simulink model "Microgrid_W"  (R2020a)
settings: Solver=ode15s  StartTime=0  StopTime=1440*1  MaxStep=1  RelTol=1e-3
libraries: simulink x4214, powerlib x685, simulink_extras x28, Microgrid_Library x18, powerlib_meascontrol x12
(part 38 of 48)

== system Microgrid_W/House 5 W1/Light 2/D10 ==
  Add : Sum  Inputs=+++
  Clock : Clock
  Compare To Zero : simulink/Logic and Bit Operations/Compare To Zero  relop=>  OutDataTypeStr=boolean
  Compare To Zero1 : simulink/Logic and Bit Operations/Compare To Zero  relop=>  OutDataTypeStr=boolean
  Compare To Zero2 : simulink/Logic and Bit Operations/Compare To Zero  relop=>  OutDataTypeStr=boolean
  Constant : Constant
  Constant{1..2,5,8} (4 alike) : Constant  Value=0
  Constant3 : Constant  Value=Dishwasher_On
  Constant4 : Constant
  Constant6 : Constant  Value=Dishwasher_On
  Constant7 : Constant
  Constant9 : Constant  Value=Dishwasher_On
  Gain : Gain  Gain=t
  Interval Test : simulink/Logic and Bit Operations/Interval Test  IntervalClosedRight=on  uplimit=Dishwasher_On+89+86400*2  IntervalClosedLeft=on  lowlimit=Dishwasher_On+82+86400*2  OutDataTypeStr=boolean
  Interval Test1 : simulink/Logic and Bit Operations/Interval Test  IntervalClosedRight=on  uplimit=Dishwasher_On+95+86400*2  IntervalClosedLeft=on  lowlimit=Dishwasher_On+90+86400*2  OutDataTypeStr=boolean
  Interval Test2 : simulink/Logic and Bit Operations/Interval Test  IntervalClosedRight=on  uplimit=Dishwasher_On+102+86400*2  IntervalClosedLeft=on  lowlimit=Dishwasher_On+97+86400*2  OutDataTypeStr=boolean
  Switch{,1..5} (6 alike) : Switch  Criteria=u2 > Threshold  Threshold=0.5
  Out1 : Outport  VectorParamsAs1DForOutWhenUnconnected=off
  wires:
  Clock/1 -> Gain/1
  Add/1 -> Out1/1
  Switch3/1 -> Add/3
  Switch2/1 -> Add/2
  Switch/1 -> Add/1
  Switch5/1 -> Switch3/1
  Switch4/1 -> Switch2/1
  Compare To Zero2/1 -> Switch5/2
  Constant8/1 -> Switch5/3
  Constant7/1 -> Switch5/1
  Constant9/1 -> Compare To Zero2/1
  Compare To Zero1/1 -> Switch4/2
  Constant5/1 -> Switch4/3
  Constant4/1 -> Switch4/1
  Constant6/1 -> Compare To Zero1/1
  Interval Test2/1 -> Switch3/2
  Interval Test1/1 -> Switch2/2
  Switch1/1 -> Switch/1
  Compare To Zero/1 -> Switch1/2
  Constant2/1 -> Switch1/3
  Constant/1 -> Switch1/1
  Constant3/1 -> Compare To Zero/1
  Gain/1 -> Interval Test/1, Interval Test1/1, Interval Test2/1
  Constant1/1 -> Switch/3, Switch2/3, Switch3/3
  Interval Test/1 -> Switch/2

== system Microgrid_W/House 5 W1/Light 2/D11 ==
  Add : Sum  Inputs=+++
  Clock : Clock
  Compare To Zero : simulink/Logic and Bit Operations/Compare To Zero  relop=>  OutDataTypeStr=boolean
  Compare To Zero1 : simulink/Logic and Bit Operations/Compare To Zero  relop=>  OutDataTypeStr=boolean
  Compare To Zero2 : simulink/Logic and Bit Operations/Compare To Zero  relop=>  OutDataTypeStr=boolean
  Constant : Constant
  Constant{1..2,5,8} (4 alike) : Constant  Value=0
  Constant3 : Constant  Value=Dishwasher_On
  Constant4 : Constant
  Constant6 : Constant  Value=Dishwasher_On
  Constant7 : Constant
  Constant9 : Constant  Value=Dishwasher_On
  Gain : Gain  Gain=t
  Interval Test : simulink/Logic and Bit Operations/Interval Test  IntervalClosedRight=on  uplimit=Dishwasher_On+89+86400*3  IntervalClosedLeft=on  lowlimit=Dishwasher_On+82+86400*3  OutDataTypeStr=boolean
  Interval Test1 : simulink/Logic and Bit Operations/Interval Test  IntervalClosedRight=on  uplimit=Dishwasher_On+95+86400*3  IntervalClosedLeft=on  lowlimit=Dishwasher_On+90+86400*3  OutDataTypeStr=boolean
  Interval Test2 : simulink/Logic and Bit Operations/Interval Test  IntervalClosedRight=on  uplimit=Dishwasher_On+102+86400*3  IntervalClosedLeft=on  lowlimit=Dishwasher_On+97+86400*3  OutDataTypeStr=boolean
  Switch{,1..5} (6 alike) : Switch  Criteria=u2 > Threshold  Threshold=0.5
  Out1 : Outport  VectorParamsAs1DForOutWhenUnconnected=off
  wires:
  Clock/1 -> Gain/1
  Interval Test/1 -> Switch/2
  Constant1/1 -> Switch3/3, Switch2/3, Switch/3
  Gain/1 -> Interval Test2/1, Interval Test1/1, Interval Test/1
  Constant3/1 -> Compare To Zero/1
  Constant/1 -> Switch1/1
  Constant2/1 -> Switch1/3
  Compare To Zero/1 -> Switch1/2
  Switch1/1 -> Switch/1
  Interval Test1/1 -> Switch2/2
  Interval Test2/1 -> Switch3/2
  Constant6/1 -> Compare To Zero1/1
  Constant4/1 -> Switch4/1
  Constant5/1 -> Switch4/3
  Compare To Zero1/1 -> Switch4/2
  Constant9/1 -> Compare To Zero2/1
  Constant7/1 -> Switch5/1
  Constant8/1 -> Switch5/3
  Compare To Zero2/1 -> Switch5/2
  Switch4/1 -> Switch2/1
  Switch5/1 -> Switch3/1
  Switch/1 -> Add/1
  Switch2/1 -> Add/2
  Switch3/1 -> Add/3
  Add/1 -> Out1/1

== system Microgrid_W/House 5 W1/Light 2/D12 ==
  Add : Sum  Inputs=+++
  Clock : Clock
  Compare To Zero : simulink/Logic and Bit Operations/Compare To Zero  relop=>  OutDataTypeStr=boolean
  Compare To Zero1 : simulink/Logic and Bit Operations/Compare To Zero  relop=>  OutDataTypeStr=boolean
  Compare To Zero2 : simulink/Logic and Bit Operations/Compare To Zero  relop=>  OutDataTypeStr=boolean
  Constant : Constant
  Constant{1..2,5,8} (4 alike) : Constant  Value=0
  Constant3 : Constant  Value=Dishwasher_On
  Constant4 : Constant
  Constant6 : Constant  Value=Dishwasher_On
  Constant7 : Constant
  Constant9 : Constant  Value=Dishwasher_On
  Gain : Gain  Gain=t
  Interval Test : simulink/Logic and Bit Operations/Interval Test  IntervalClosedRight=on  uplimit=Dishwasher_On+89+86400*4  IntervalClosedLeft=on  lowlimit=Dishwasher_On+82+86400*4  OutDataTypeStr=boolean
  Interval Test1 : simulink/Logic and Bit Operations/Interval Test  IntervalClosedRight=on  uplimit=Dishwasher_On+95+86400*4  IntervalClosedLeft=on  lowlimit=Dishwasher_On+90+86400*4  OutDataTypeStr=boolean
  Interval Test2 : simulink/Logic and Bit Operations/Interval Test  IntervalClosedRight=on  uplimit=Dishwasher_On+102+86400*4  IntervalClosedLeft=on  lowlimit=Dishwasher_On+97+86400*4  OutDataTypeStr=boolean
  Switch{,1..5} (6 alike) : Switch  Criteria=u2 > Threshold  Threshold=0.5
  Out1 : Outport  VectorParamsAs1DForOutWhenUnconnected=off
  wires:
  Clock/1 -> Gain/1
  Add/1 -> Out1/1
  Switch3/1 -> Add/3
  Switch2/1 -> Add/2
  Switch/1 -> Add/1
  Switch5/1 -> Switch3/1
  Switch4/1 -> Switch2/1
  Compare To Zero2/1 -> Switch5/2
  Constant8/1 -> Switch5/3
  Constant7/1 -> Switch5/1
  Constant9/1 -> Compare To Zero2/1
  Compare To Zero1/1 -> Switch4/2
  Constant5/1 -> Switch4/3
  Constant4/1 -> Switch4/1
  Constant6/1 -> Compare To Zero1/1
  Interval Test2/1 -> Switch3/2
  Interval Test1/1 -> Switch2/2
  Switch1/1 -> Switch/1
  Compare To Zero/1 -> Switch1/2
  Constant2/1 -> Switch1/3
  Constant/1 -> Switch1/1
  Constant3/1 -> Compare To Zero/1
  Gain/1 -> Interval Test/1, Interval Test1/1, Interval Test2/1
  Constant1/1 -> Switch/3, Switch2/3, Switch3/3
  Interval Test/1 -> Switch/2

== system Microgrid_W/House 5 W1/Light 2/D13 ==
  Add : Sum  Inputs=+++
  Clock : Clock
  Compare To Zero : simulink/Logic and Bit Operations/Compare To Zero  relop=>  OutDataTypeStr=boolean
  Compare To Zero1 : simulink/Logic and Bit Operations/Compare To Zero  relop=>  OutDataTypeStr=boolean
  Compare To Zero2 : simulink/Logic and Bit Operations/Compare To Zero  relop=>  OutDataTypeStr=boolean
  Constant : Constant
  Constant{1..2,5,8} (4 alike) : Constant  Value=0
  Constant3 : Constant  Value=Dishwasher_On
  Constant4 : Constant
  Constant6 : Constant  Value=Dishwasher_On
  Constant7 : Constant
  Constant9 : Constant  Value=Dishwasher_On
  Gain : Gain  Gain=t
  Interval Test : simulink/Logic and Bit Operations/Interval Test  IntervalClosedRight=on  uplimit=Dishwasher_On+89+86400*5  IntervalClosedLeft=on  lowlimit=Dishwasher_On+82+86400*5  OutDataTypeStr=boolean
  Interval Test1 : simulink/Logic and Bit Operations/Interval Test  IntervalClosedRight=on  uplimit=Dishwasher_On+95+86400*5  IntervalClosedLeft=on  lowlimit=Dishwasher_On+90+86400*5  OutDataTypeStr=boolean
  Interval Test2 : simulink/Logic and Bit Operations/Interval Test  IntervalClosedRight=on  uplimit=Dishwasher_On+102+86400*5  IntervalClosedLeft=on  lowlimit=Dishwasher_On+97+86400*5  OutDataTypeStr=boolean
  Switch{,1..5} (6 alike) : Switch  Criteria=u2 > Threshold  Threshold=0.5
  Out1 : Outport  VectorParamsAs1DForOutWhenUnconnected=off
  wires:
  Clock/1 -> Gain/1
  Interval Test/1 -> Switch/2
  Constant1/1 -> Switch3/3, Switch2/3, Switch/3
  Gain/1 -> Interval Test2/1, Interval Test1/1, Interval Test/1
  Constant3/1 -> Compare To Zero/1
  Constant/1 -> Switch1/1
  Constant2/1 -> Switch1/3
  Compare To Zero/1 -> Switch1/2
  Switch1/1 -> Switch/1
  Interval Test1/1 -> Switch2/2
  Interval Test2/1 -> Switch3/2
  Constant6/1 -> Compare To Zero1/1
  Constant4/1 -> Switch4/1
  Constant5/1 -> Switch4/3
  Compare To Zero1/1 -> Switch4/2
  Constant9/1 -> Compare To Zero2/1
  Constant7/1 -> Switch5/1
  Constant8/1 -> Switch5/3
  Compare To Zero2/1 -> Switch5/2
  Switch4/1 -> Switch2/1
  Switch5/1 -> Switch3/1
  Switch/1 -> Add/1
  Switch2/1 -> Add/2
  Switch3/1 -> Add/3
  Add/1 -> Out1/1

== system Microgrid_W/House 5 W1/Light 2/D14 ==
  Add : Sum  Inputs=+++
  Clock : Clock
  Compare To Zero : simulink/Logic and Bit Operations/Compare To Zero  relop=>  OutDataTypeStr=boolean
  Compare To Zero1 : simulink/Logic and Bit Operations/Compare To Zero  relop=>  OutDataTypeStr=boolean
  Compare To Zero2 : simulink/Logic and Bit Operations/Compare To Zero  relop=>  OutDataTypeStr=boolean
  Constant : Constant
  Constant{1..2,5,8} (4 alike) : Constant  Value=0
  Constant3 : Constant  Value=Dishwasher_On
  Constant4 : Constant
  Constant6 : Constant  Value=Dishwasher_On
  Constant7 : Constant
  Constant9 : Constant  Value=Dishwasher_On
  Gain : Gain  Gain=t
  Interval Test : simulink/Logic and Bit Operations/Interval Test  IntervalClosedRight=on  uplimit=Dishwasher_On+89+86400*6  IntervalClosedLeft=on  lowlimit=Dishwasher_On+82+86400*6  OutDataTypeStr=boolean
  Interval Test1 : simulink/Logic and Bit Operations/Interval Test  IntervalClosedRight=on  uplimit=Dishwasher_On+95+86400*6  IntervalClosedLeft=on  lowlimit=Dishwasher_On+90+86400*6  OutDataTypeStr=boolean
  Interval Test2 : simulink/Logic and Bit Operations/Interval Test  IntervalClosedRight=on  uplimit=Dishwasher_On+102+86400*6  IntervalClosedLeft=on  lowlimit=Dishwasher_On+97+86400*6  OutDataTypeStr=boolean
  Switch{,1..5} (6 alike) : Switch  Criteria=u2 > Threshold  Threshold=0.5
  Out1 : Outport  VectorParamsAs1DForOutWhenUnconnected=off
  wires:
  Clock/1 -> Gain/1
  Add/1 -> Out1/1
  Switch3/1 -> Add/3
  Switch2/1 -> Add/2
  Switch/1 -> Add/1
  Switch5/1 -> Switch3/1
  Switch4/1 -> Switch2/1
  Compare To Zero2/1 -> Switch5/2
  Constant8/1 -> Switch5/3
  Constant7/1 -> Switch5/1
  Constant9/1 -> Compare To Zero2/1
  Compare To Zero1/1 -> Switch4/2
  Constant5/1 -> Switch4/3
  Constant4/1 -> Switch4/1
  Constant6/1 -> Compare To Zero1/1
  Interval Test2/1 -> Switch3/2
  Interval Test1/1 -> Switch2/2
  Switch1/1 -> Switch/1
  Compare To Zero/1 -> Switch1/2
  Constant2/1 -> Switch1/3
  Constant/1 -> Switch1/1
  Constant3/1 -> Compare To Zero/1
  Gain/1 -> Interval Test/1, Interval Test1/1, Interval Test2/1
  Constant1/1 -> Switch/3, Switch2/3, Switch3/3
  Interval Test/1 -> Switch/2

== system Microgrid_W/House 5 W1/Light 2/D15 ==
  Add : Sum  Inputs=+++
  Clock : Clock
  Compare To Zero : simulink/Logic and Bit Operations/Compare To Zero  relop=>  OutDataTypeStr=boolean
  Compare To Zero1 : simulink/Logic and Bit Operations/Compare To Zero  relop=>  OutDataTypeStr=boolean
  Compare To Zero2 : simulink/Logic and Bit Operations/Compare To Zero  relop=>  OutDataTypeStr=boolean
  Constant : Constant
  Constant{1..2,5,8} (4 alike) : Constant  Value=0
  Constant3 : Constant  Value=Dishwasher_On
  Constant4 : Constant
  Constant6 : Constant  Value=Dishwasher_On
  Constant7 : Constant
  Constant9 : Constant  Value=Dishwasher_On
  Gain : Gain  Gain=t
  Interval Test : simulink/Logic and Bit Operations/Interval Test  IntervalClosedRight=on  uplimit=Dishwasher_On+10  IntervalClosedLeft=on  lowlimit=Dishwasher_On  OutDataTypeStr=boolean
  Interval Test1 : simulink/Logic and Bit Operations/Interval Test  IntervalClosedRight=on  uplimit=Dishwasher_On+48  IntervalClosedLeft=on  lowlimit=Dishwasher_On+23  OutDataTypeStr=boolean
  Interval Test2 : simulink/Logic and Bit Operations/Interval Test  IntervalClosedRight=on  uplimit=Dishwasher_On+75  IntervalClosedLeft=on  lowlimit=Dishwasher_On+66  OutDataTypeStr=boolean
  Switch{,1..5} (6 alike) : Switch  Criteria=u2 > Threshold  Threshold=0.5
  Out1 : Outport  VectorParamsAs1DForOutWhenUnconnected=off
  wires:
  Clock/1 -> Gain/1
  Interval Test/1 -> Switch/2
  Constant1/1 -> Switch3/3, Switch2/3, Switch/3
  Gain/1 -> Interval Test2/1, Interval Test1/1, Interval Test/1
  Constant3/1 -> Compare To Zero/1
  Constant/1 -> Switch1/1
  Constant2/1 -> Switch1/3
  Compare To Zero/1 -> Switch1/2
  Switch1/1 -> Switch/1
  Interval Test1/1 -> Switch2/2
  Interval Test2/1 -> Switch3/2
  Constant6/1 -> Compare To Zero1/1
  Constant4/1 -> Switch4/1
  Constant5/1 -> Switch4/3
  Compare To Zero1/1 -> Switch4/2
  Constant9/1 -> Compare To Zero2/1
  Constant7/1 -> Switch5/1
  Constant8/1 -> Switch5/3
  Compare To Zero2/1 -> Switch5/2
  Switch4/1 -> Switch2/1
  Switch5/1 -> Switch3/1
  Switch/1 -> Add/1
  Switch2/1 -> Add/2
  Switch3/1 -> Add/3
  Add/1 -> Out1/1

== system Microgrid_W/House 5 W1/Light 2/D16 ==
  Add : Sum  Inputs=+++
  Clock : Clock
  Compare To Zero : simulink/Logic and Bit Operations/Compare To Zero  relop=>  OutDataTypeStr=boolean
  Compare To Zero1 : simulink/Logic and Bit Operations/Compare To Zero  relop=>  OutDataTypeStr=boolean
  Compare To Zero2 : simulink/Logic and Bit Operations/Compare To Zero  relop=>  OutDataTypeStr=boolean
  Constant : Constant
  Constant{1..2,5,8} (4 alike) : Constant  Value=0
  Constant3 : Constant  Value=Dishwasher_On
  Constant4 : Constant
  Constant6 : Constant  Value=Dishwasher_On
  Constant7 : Constant
  Constant9 : Constant  Value=Dishwasher_On
  Gain : Gain  Gain=t
  Interval Test : simulink/Logic and Bit Operations/Interval Test  IntervalClosedRight=on  uplimit=Dishwasher_On+10+86400  IntervalClosedLeft=on  lowlimit=Dishwasher_On+86400  OutDataTypeStr=boolean
  Interval Test1 : simulink/Logic and Bit Operations/Interval Test  IntervalClosedRight=on  uplimit=Dishwasher_On+48+86400  IntervalClosedLeft=on  lowlimit=Dishwasher_On+23+86400  OutDataTypeStr=boolean
  Interval Test2 : simulink/Logic and Bit Operations/Interval Test  IntervalClosedRight=on  uplimit=Dishwasher_On+75+86400  IntervalClosedLeft=on  lowlimit=Dishwasher_On+66+86400  OutDataTypeStr=boolean
  Switch{,1..5} (6 alike) : Switch  Criteria=u2 > Threshold  Threshold=0.5
  Out1 : Outport  VectorParamsAs1DForOutWhenUnconnected=off
  wires:
  Clock/1 -> Gain/1
  Add/1 -> Out1/1
  Switch3/1 -> Add/3
  Switch2/1 -> Add/2
  Switch/1 -> Add/1
  Switch5/1 -> Switch3/1
  Switch4/1 -> Switch2/1
  Compare To Zero2/1 -> Switch5/2
  Constant8/1 -> Switch5/3
  Constant7/1 -> Switch5/1
  Constant9/1 -> Compare To Zero2/1
  Compare To Zero1/1 -> Switch4/2
  Constant5/1 -> Switch4/3
  Constant4/1 -> Switch4/1
  Constant6/1 -> Compare To Zero1/1
  Interval Test2/1 -> Switch3/2
  Interval Test1/1 -> Switch2/2
  Switch1/1 -> Switch/1
  Compare To Zero/1 -> Switch1/2
  Constant2/1 -> Switch1/3
  Constant/1 -> Switch1/1
  Constant3/1 -> Compare To Zero/1
  Gain/1 -> Interval Test/1, Interval Test1/1, Interval Test2/1
  Constant1/1 -> Switch/3, Switch2/3, Switch3/3
  Interval Test/1 -> Switch/2

== system Microgrid_W/House 5 W1/Light 2/D17 ==
  Add : Sum  Inputs=+++
  Clock : Clock
  Compare To Zero : simulink/Logic and Bit Operations/Compare To Zero  relop=>  OutDataTypeStr=boolean
  Compare To Zero1 : simulink/Logic and Bit Operations/Compare To Zero  relop=>  OutDataTypeStr=boolean
  Compare To Zero2 : simulink/Logic and Bit Operations/Compare To Zero  relop=>  OutDataTypeStr=boolean
  Constant : Constant
  Constant{1..2,5,8} (4 alike) : Constant  Value=0
  Constant3 : Constant  Value=Dishwasher_On
  Constant4 : Constant
  Constant6 : Constant  Value=Dishwasher_On
  Constant7 : Constant
  Constant9 : Constant  Value=Dishwasher_On
  Gain : Gain  Gain=t
  Interval Test : simulink/Logic and Bit Operations/Interval Test  IntervalClosedRight=on  uplimit=Dishwasher_On+10+86400*2  IntervalClosedLeft=on  lowlimit=Dishwasher_On+86400*2  OutDataTypeStr=boolean
  Interval Test1 : simulink/Logic and Bit Operations/Interval Test  IntervalClosedRight=on  uplimit=Dishwasher_On+48+86400*2  IntervalClosedLeft=on  lowlimit=Dishwasher_On+23+86400*2  OutDataTypeStr=boolean
  Interval Test2 : simulink/Logic and Bit Operations/Interval Test  IntervalClosedRight=on  uplimit=Dishwasher_On+75+86400*2  IntervalClosedLeft=on  lowlimit=Dishwasher_On+66+86400*2  OutDataTypeStr=boolean
  Switch{,1..5} (6 alike) : Switch  Criteria=u2 > Threshold  Threshold=0.5
  Out1 : Outport  VectorParamsAs1DForOutWhenUnconnected=off
  wires:
  Clock/1 -> Gain/1
  Interval Test/1 -> Switch/2
  Constant1/1 -> Switch3/3, Switch2/3, Switch/3
  Gain/1 -> Interval Test2/1, Interval Test1/1, Interval Test/1
  Constant3/1 -> Compare To Zero/1
  Constant/1 -> Switch1/1
  Constant2/1 -> Switch1/3
  Compare To Zero/1 -> Switch1/2
  Switch1/1 -> Switch/1
  Interval Test1/1 -> Switch2/2
  Interval Test2/1 -> Switch3/2
  Constant6/1 -> Compare To Zero1/1
  Constant4/1 -> Switch4/1
  Constant5/1 -> Switch4/3
  Compare To Zero1/1 -> Switch4/2
  Constant9/1 -> Compare To Zero2/1
  Constant7/1 -> Switch5/1
  Constant8/1 -> Switch5/3
  Compare To Zero2/1 -> Switch5/2
  Switch4/1 -> Switch2/1
  Switch5/1 -> Switch3/1
  Switch/1 -> Add/1
  Switch2/1 -> Add/2
  Switch3/1 -> Add/3
  Add/1 -> Out1/1

== system Microgrid_W/House 5 W1/Light 2/D18 ==
  Add : Sum  Inputs=+++
  Clock : Clock
  Compare To Zero : simulink/Logic and Bit Operations/Compare To Zero  relop=>  OutDataTypeStr=boolean
  Compare To Zero1 : simulink/Logic and Bit Operations/Compare To Zero  relop=>  OutDataTypeStr=boolean
  Compare To Zero2 : simulink/Logic and Bit Operations/Compare To Zero  relop=>  OutDataTypeStr=boolean
  Constant : Constant
  Constant{1..2,5,8} (4 alike) : Constant  Value=0
  Constant3 : Constant  Value=Dishwasher_On
  Constant4 : Constant
  Constant6 : Constant  Value=Dishwasher_On
  Constant7 : Constant
  Constant9 : Constant  Value=Dishwasher_On
  Gain : Gain  Gain=t
  Interval Test : simulink/Logic and Bit Operations/Interval Test  IntervalClosedRight=on  uplimit=Dishwasher_On+10+86400*3  IntervalClosedLeft=on  lowlimit=Dishwasher_On+86400*3  OutDataTypeStr=boolean
  Interval Test1 : simulink/Logic and Bit Operations/Interval Test  IntervalClosedRight=on  uplimit=Dishwasher_On+48+86400*3  IntervalClosedLeft=on  lowlimit=Dishwasher_On+23+86400*3  OutDataTypeStr=boolean
  Interval Test2 : simulink/Logic and Bit Operations/Interval Test  IntervalClosedRight=on  uplimit=Dishwasher_On+75+86400*3  IntervalClosedLeft=on  lowlimit=Dishwasher_On+66+86400*3  OutDataTypeStr=boolean
  Switch{,1..5} (6 alike) : Switch  Criteria=u2 > Threshold  Threshold=0.5
  Out1 : Outport  VectorParamsAs1DForOutWhenUnconnected=off
  wires:
  Clock/1 -> Gain/1
  Add/1 -> Out1/1
  Switch3/1 -> Add/3
  Switch2/1 -> Add/2
  Switch/1 -> Add/1
  Switch5/1 -> Switch3/1
  Switch4/1 -> Switch2/1
  Compare To Zero2/1 -> Switch5/2
  Constant8/1 -> Switch5/3
  Constant7/1 -> Switch5/1
  Constant9/1 -> Compare To Zero2/1
  Compare To Zero1/1 -> Switch4/2
  Constant5/1 -> Switch4/3
  Constant4/1 -> Switch4/1
  Constant6/1 -> Compare To Zero1/1
  Interval Test2/1 -> Switch3/2
  Interval Test1/1 -> Switch2/2
  Switch1/1 -> Switch/1
  Compare To Zero/1 -> Switch1/2
  Constant2/1 -> Switch1/3
  Constant/1 -> Switch1/1
  Constant3/1 -> Compare To Zero/1
  Gain/1 -> Interval Test/1, Interval Test1/1, Interval Test2/1
  Constant1/1 -> Switch/3, Switch2/3, Switch3/3
  Interval Test/1 -> Switch/2

== system Microgrid_W/House 5 W1/Light 2/D19 ==
  Add : Sum  Inputs=+++
  Clock : Clock
  Compare To Zero : simulink/Logic and Bit Operations/Compare To Zero  relop=>  OutDataTypeStr=boolean
  Compare To Zero1 : simulink/Logic and Bit Operations/Compare To Zero  relop=>  OutDataTypeStr=boolean
  Compare To Zero2 : simulink/Logic and Bit Operations/Compare To Zero  relop=>  OutDataTypeStr=boolean
  Constant : Constant
  Constant{1..2,5,8} (4 alike) : Constant  Value=0
  Constant3 : Constant  Value=Dishwasher_On
  Constant4 : Constant
  Constant6 : Constant  Value=Dishwasher_On
  Constant7 : Constant
  Constant9 : Constant  Value=Dishwasher_On
  Gain : Gain  Gain=t
  Interval Test : simulink/Logic and Bit Operations/Interval Test  IntervalClosedRight=on  uplimit=Dishwasher_On+10+86400*4  IntervalClosedLeft=on  lowlimit=Dishwasher_On+86400*4  OutDataTypeStr=boolean
  Interval Test1 : simulink/Logic and Bit Operations/Interval Test  IntervalClosedRight=on  uplimit=Dishwasher_On+48+86400*4  IntervalClosedLeft=on  lowlimit=Dishwasher_On+23+86400*4  OutDataTypeStr=boolean
  Interval Test2 : simulink/Logic and Bit Operations/Interval Test  IntervalClosedRight=on  uplimit=Dishwasher_On+75+86400*4  IntervalClosedLeft=on  lowlimit=Dishwasher_On+66+86400*4  OutDataTypeStr=boolean
  Switch{,1..5} (6 alike) : Switch  Criteria=u2 > Threshold  Threshold=0.5
  Out1 : Outport  VectorParamsAs1DForOutWhenUnconnected=off
  wires:
  Clock/1 -> Gain/1
  Interval Test/1 -> Switch/2
  Constant1/1 -> Switch3/3, Switch2/3, Switch/3
  Gain/1 -> Interval Test2/1, Interval Test1/1, Interval Test/1
  Constant3/1 -> Compare To Zero/1
  Constant/1 -> Switch1/1
  Constant2/1 -> Switch1/3
  Compare To Zero/1 -> Switch1/2
  Switch1/1 -> Switch/1
  Interval Test1/1 -> Switch2/2
  Interval Test2/1 -> Switch3/2
  Constant6/1 -> Compare To Zero1/1
  Constant4/1 -> Switch4/1
  Constant5/1 -> Switch4/3
  Compare To Zero1/1 -> Switch4/2
  Constant9/1 -> Compare To Zero2/1
  Constant7/1 -> Switch5/1
  Constant8/1 -> Switch5/3
  Compare To Zero2/1 -> Switch5/2
  Switch4/1 -> Switch2/1
  Switch5/1 -> Switch3/1
  Switch/1 -> Add/1
  Switch2/1 -> Add/2
  Switch3/1 -> Add/3
  Add/1 -> Out1/1

== system Microgrid_W/House 5 W1/Light 2/D2 ==
  Add : Sum
  Clock : Clock
  Compare To Zero : simulink/Logic and Bit Operations/Compare To Zero  relop=>  OutDataTypeStr=boolean
  Compare To Zero1 : simulink/Logic and Bit Operations/Compare To Zero  relop=>  OutDataTypeStr=boolean
  Constant : Constant
  Constant1 : Constant  Value=0
  Constant2 : Constant  Value=0
  Constant3 : Constant  Value=Dishwasher_On
  Constant4 : Constant
  Constant5 : Constant  Value=0
  Constant6 : Constant  Value=Dishwasher_On
  Gain : Gain  Gain=t
  Interval Test : simulink/Logic and Bit Operations/Interval Test  IntervalClosedRight=on  uplimit=Dishwasher_On+23+86400  IntervalClosedLeft=on  lowlimit=Dishwasher_On+13+86400  OutDataTypeStr=boolean
  Interval Test1 : simulink/Logic and Bit Operations/Interval Test  IntervalClosedRight=on  uplimit=Dishwasher_On+66+86400  IntervalClosedLeft=on  lowlimit=Dishwasher_On+52+86400  OutDataTypeStr=boolean
  Switch{,1..2,4} (4 alike) : Switch  Criteria=u2 > Threshold  Threshold=0.5
  Out1 : Outport  VectorParamsAs1DForOutWhenUnconnected=off
  wires:
  Clock/1 -> Gain/1
  Interval Test/1 -> Switch/2
  Constant1/1 -> Switch2/3, Switch/3
  Gain/1 -> Interval Test/1, Interval Test1/1
  Constant3/1 -> Compare To Zero/1
  Constant/1 -> Switch1/1
  Constant2/1 -> Switch1/3
  Compare To Zero/1 -> Switch1/2
  Switch1/1 -> Switch/1
  Interval Test1/1 -> Switch2/2
  Constant6/1 -> Compare To Zero1/1
  Constant4/1 -> Switch4/1
  Constant5/1 -> Switch4/3
  Compare To Zero1/1 -> Switch4/2
  Switch4/1 -> Switch2/1
  Switch/1 -> Add/1
  Switch2/1 -> Add/2
  Add/1 -> Out1/1

== system Microgrid_W/House 5 W1/Light 2/D20 ==
  Add : Sum  Inputs=+++
  Clock : Clock
  Compare To Zero : simulink/Logic and Bit Operations/Compare To Zero  relop=>  OutDataTypeStr=boolean
  Compare To Zero1 : simulink/Logic and Bit Operations/Compare To Zero  relop=>  OutDataTypeStr=boolean
  Compare To Zero2 : simulink/Logic and Bit Operations/Compare To Zero  relop=>  OutDataTypeStr=boolean
  Constant : Constant
  Constant{1..2,5,8} (4 alike) : Constant  Value=0
  Constant3 : Constant  Value=Dishwasher_On
  Constant4 : Constant
  Constant6 : Constant  Value=Dishwasher_On
  Constant7 : Constant
  Constant9 : Constant  Value=Dishwasher_On
  Gain : Gain  Gain=t
  Interval Test : simulink/Logic and Bit Operations/Interval Test  IntervalClosedRight=on  uplimit=Dishwasher_On+10+86400*5  IntervalClosedLeft=on  lowlimit=Dishwasher_On+86400*5  OutDataTypeStr=boolean
  Interval Test1 : simulink/Logic and Bit Operations/Interval Test  IntervalClosedRight=on  uplimit=Dishwasher_On+48+86400*5  IntervalClosedLeft=on  lowlimit=Dishwasher_On+23+86400*5  OutDataTypeStr=boolean
  Interval Test2 : simulink/Logic and Bit Operations/Interval Test  IntervalClosedRight=on  uplimit=Dishwasher_On+75+86400*5  IntervalClosedLeft=on  lowlimit=Dishwasher_On+66+86400*5  OutDataTypeStr=boolean
  Switch{,1..5} (6 alike) : Switch  Criteria=u2 > Threshold  Threshold=0.5
  Out1 : Outport  VectorParamsAs1DForOutWhenUnconnected=off
  wires:
  Clock/1 -> Gain/1
  Add/1 -> Out1/1
  Switch3/1 -> Add/3
  Switch2/1 -> Add/2
  Switch/1 -> Add/1
  Switch5/1 -> Switch3/1
  Switch4/1 -> Switch2/1
  Compare To Zero2/1 -> Switch5/2
  Constant8/1 -> Switch5/3
  Constant7/1 -> Switch5/1
  Constant9/1 -> Compare To Zero2/1
  Compare To Zero1/1 -> Switch4/2
  Constant5/1 -> Switch4/3
  Constant4/1 -> Switch4/1
  Constant6/1 -> Compare To Zero1/1
  Interval Test2/1 -> Switch3/2
  Interval Test1/1 -> Switch2/2
  Switch1/1 -> Switch/1
  Compare To Zero/1 -> Switch1/2
  Constant2/1 -> Switch1/3
  Constant/1 -> Switch1/1
  Constant3/1 -> Compare To Zero/1
  Gain/1 -> Interval Test/1, Interval Test1/1, Interval Test2/1
  Constant1/1 -> Switch/3, Switch2/3, Switch3/3
  Interval Test/1 -> Switch/2

== system Microgrid_W/House 5 W1/Light 2/D21 ==
  Add : Sum  Inputs=+++
  Clock : Clock
  Compare To Zero : simulink/Logic and Bit Operations/Compare To Zero  relop=>  OutDataTypeStr=boolean
  Compare To Zero1 : simulink/Logic and Bit Operations/Compare To Zero  relop=>  OutDataTypeStr=boolean
  Compare To Zero2 : simulink/Logic and Bit Operations/Compare To Zero  relop=>  OutDataTypeStr=boolean
  Constant : Constant
  Constant{1..2,5,8} (4 alike) : Constant  Value=0
  Constant3 : Constant  Value=Dishwasher_On
  Constant4 : Constant
  Constant6 : Constant  Value=Dishwasher_On
  Constant7 : Constant
  Constant9 : Constant  Value=Dishwasher_On
  Gain : Gain  Gain=t
  Interval Test : simulink/Logic and Bit Operations/Interval Test  IntervalClosedRight=on  uplimit=Dishwasher_On+10+86400*6  IntervalClosedLeft=on  lowlimit=Dishwasher_On+86400*6  OutDataTypeStr=boolean
  Interval Test1 : simulink/Logic and Bit Operations/Interval Test  IntervalClosedRight=on  uplimit=Dishwasher_On+48+86400*6  IntervalClosedLeft=on  lowlimit=Dishwasher_On+23+86400*6  OutDataTypeStr=boolean
  Interval Test2 : simulink/Logic and Bit Operations/Interval Test  IntervalClosedRight=on  uplimit=Dishwasher_On+75+86400*6  IntervalClosedLeft=on  lowlimit=Dishwasher_On+66+86400*6  OutDataTypeStr=boolean
  Switch{,1..5} (6 alike) : Switch  Criteria=u2 > Threshold  Threshold=0.5
  Out1 : Outport  VectorParamsAs1DForOutWhenUnconnected=off
  wires:
  Clock/1 -> Gain/1
  Interval Test/1 -> Switch/2
  Constant1/1 -> Switch3/3, Switch2/3, Switch/3
  Gain/1 -> Interval Test2/1, Interval Test1/1, Interval Test/1
  Constant3/1 -> Compare To Zero/1
  Constant/1 -> Switch1/1
  Constant2/1 -> Switch1/3
  Compare To Zero/1 -> Switch1/2
  Switch1/1 -> Switch/1
  Interval Test1/1 -> Switch2/2
  Interval Test2/1 -> Switch3/2
  Constant6/1 -> Compare To Zero1/1
  Constant4/1 -> Switch4/1
  Constant5/1 -> Switch4/3
  Compare To Zero1/1 -> Switch4/2
  Constant9/1 -> Compare To Zero2/1
  Constant7/1 -> Switch5/1
  Constant8/1 -> Switch5/3
  Compare To Zero2/1 -> Switch5/2
  Switch4/1 -> Switch2/1
  Switch5/1 -> Switch3/1
  Switch/1 -> Add/1
  Switch2/1 -> Add/2
  Switch3/1 -> Add/3
  Add/1 -> Out1/1

== system Microgrid_W/House 5 W1/Light 2/D3 ==
  Add : Sum
  Clock : Clock
  Compare To Zero : simulink/Logic and Bit Operations/Compare To Zero  relop=>  OutDataTypeStr=boolean
  Compare To Zero1 : simulink/Logic and Bit Operations/Compare To Zero  relop=>  OutDataTypeStr=boolean
  Constant : Constant
  Constant1 : Constant  Value=0
  Constant2 : Constant  Value=0
  Constant3 : Constant  Value=Dishwasher_On
  Constant4 : Constant
  Constant5 : Constant  Value=0
  Constant6 : Constant  Value=Dishwasher_On
  Gain : Gain  Gain=t
  Interval Test : simulink/Logic and Bit Operations/Interval Test  IntervalClosedRight=on  uplimit=Dishwasher_On+23+86400*2  IntervalClosedLeft=on  lowlimit=Dishwasher_On+13+86400*2  OutDataTypeStr=boolean
  Interval Test1 : simulink/Logic and Bit Operations/Interval Test  IntervalClosedRight=on  uplimit=Dishwasher_On+66+86400*2  IntervalClosedLeft=on  lowlimit=Dishwasher_On+52+86400*2  OutDataTypeStr=boolean
  Switch{,1..2,4} (4 alike) : Switch  Criteria=u2 > Threshold  Threshold=0.5
  Out1 : Outport  VectorParamsAs1DForOutWhenUnconnected=off
  wires:
  Clock/1 -> Gain/1
  Add/1 -> Out1/1
  Switch2/1 -> Add/2
  Switch/1 -> Add/1
  Switch4/1 -> Switch2/1
  Compare To Zero1/1 -> Switch4/2
  Constant5/1 -> Switch4/3
  Constant4/1 -> Switch4/1
  Constant6/1 -> Compare To Zero1/1
  Interval Test1/1 -> Switch2/2
  Switch1/1 -> Switch/1
  Compare To Zero/1 -> Switch1/2
  Constant2/1 -> Switch1/3
  Constant/1 -> Switch1/1
  Constant3/1 -> Compare To Zero/1
  Gain/1 -> Interval Test1/1, Interval Test/1
  Constant1/1 -> Switch/3, Switch2/3
  Interval Test/1 -> Switch/2

== system Microgrid_W/House 5 W1/Light 2/D4 ==
  Add : Sum
  Clock : Clock
  Compare To Zero : simulink/Logic and Bit Operations/Compare To Zero  relop=>  OutDataTypeStr=boolean
  Compare To Zero1 : simulink/Logic and Bit Operations/Compare To Zero  relop=>  OutDataTypeStr=boolean
  Constant : Constant
  Constant1 : Constant  Value=0
  Constant2 : Constant  Value=0
  Constant3 : Constant  Value=Dishwasher_On
  Constant4 : Constant
  Constant5 : Constant  Value=0
  Constant6 : Constant  Value=Dishwasher_On
  Gain : Gain  Gain=t
  Interval Test : simulink/Logic and Bit Operations/Interval Test  IntervalClosedRight=on  uplimit=Dishwasher_On+23+86400*3  IntervalClosedLeft=on  lowlimit=Dishwasher_On+13+86400*3  OutDataTypeStr=boolean
  Interval Test1 : simulink/Logic and Bit Operations/Interval Test  IntervalClosedRight=on  uplimit=Dishwasher_On+66+86400*3  IntervalClosedLeft=on  lowlimit=Dishwasher_On+52+86400*3  OutDataTypeStr=boolean
  Switch{,1..2,4} (4 alike) : Switch  Criteria=u2 > Threshold  Threshold=0.5
  Out1 : Outport  VectorParamsAs1DForOutWhenUnconnected=off
  wires:
  Clock/1 -> Gain/1
  Interval Test/1 -> Switch/2
  Constant1/1 -> Switch2/3, Switch/3
  Gain/1 -> Interval Test/1, Interval Test1/1
  Constant3/1 -> Compare To Zero/1
  Constant/1 -> Switch1/1
  Constant2/1 -> Switch1/3
  Compare To Zero/1 -> Switch1/2
  Switch1/1 -> Switch/1
  Interval Test1/1 -> Switch2/2
  Constant6/1 -> Compare To Zero1/1
  Constant4/1 -> Switch4/1
  Constant5/1 -> Switch4/3
  Compare To Zero1/1 -> Switch4/2
  Switch4/1 -> Switch2/1
  Switch/1 -> Add/1
  Switch2/1 -> Add/2
  Add/1 -> Out1/1

== system Microgrid_W/House 5 W1/Light 2/D5 ==
  Add : Sum
  Clock : Clock
  Compare To Zero : simulink/Logic and Bit Operations/Compare To Zero  relop=>  OutDataTypeStr=boolean
  Compare To Zero1 : simulink/Logic and Bit Operations/Compare To Zero  relop=>  OutDataTypeStr=boolean
  Constant : Constant
  Constant1 : Constant  Value=0
  Constant2 : Constant  Value=0
  Constant3 : Constant  Value=Dishwasher_On
  Constant4 : Constant
  Constant5 : Constant  Value=0
  Constant6 : Constant  Value=Dishwasher_On
  Gain : Gain  Gain=t
  Interval Test : simulink/Logic and Bit Operations/Interval Test  IntervalClosedRight=on  uplimit=Dishwasher_On+23+86400*4  IntervalClosedLeft=on  lowlimit=Dishwasher_On+13+86400*4  OutDataTypeStr=boolean
  Interval Test1 : simulink/Logic and Bit Operations/Interval Test  IntervalClosedRight=on  uplimit=Dishwasher_On+66+86400*4  IntervalClosedLeft=on  lowlimit=Dishwasher_On+52+86400*4  OutDataTypeStr=boolean
  Switch{,1..2,4} (4 alike) : Switch  Criteria=u2 > Threshold  Threshold=0.5
  Out1 : Outport  VectorParamsAs1DForOutWhenUnconnected=off
  wires:
  Clock/1 -> Gain/1
  Add/1 -> Out1/1
  Switch2/1 -> Add/2
  Switch/1 -> Add/1
  Switch4/1 -> Switch2/1
  Compare To Zero1/1 -> Switch4/2
  Constant5/1 -> Switch4/3
  Constant4/1 -> Switch4/1
  Constant6/1 -> Compare To Zero1/1
  Interval Test1/1 -> Switch2/2
  Switch1/1 -> Switch/1
  Compare To Zero/1 -> Switch1/2
  Constant2/1 -> Switch1/3
  Constant/1 -> Switch1/1
  Constant3/1 -> Compare To Zero/1
  Gain/1 -> Interval Test1/1, Interval Test/1
  Constant1/1 -> Switch/3, Switch2/3
  Interval Test/1 -> Switch/2

== system Microgrid_W/House 5 W1/Light 2/D6 ==
  Add : Sum
  Clock : Clock
  Compare To Zero : simulink/Logic and Bit Operations/Compare To Zero  relop=>  OutDataTypeStr=boolean
  Compare To Zero1 : simulink/Logic and Bit Operations/Compare To Zero  relop=>  OutDataTypeStr=boolean
  Constant : Constant
  Constant1 : Constant  Value=0
  Constant2 : Constant  Value=0
  Constant3 : Constant  Value=Dishwasher_On
  Constant4 : Constant
  Constant5 : Constant  Value=0
  Constant6 : Constant  Value=Dishwasher_On
  Gain : Gain  Gain=t
  Interval Test : simulink/Logic and Bit Operations/Interval Test  IntervalClosedRight=on  uplimit=Dishwasher_On+23+86400*5  IntervalClosedLeft=on  lowlimit=Dishwasher_On+13+86400*5  OutDataTypeStr=boolean
  Interval Test1 : simulink/Logic and Bit Operations/Interval Test  IntervalClosedRight=on  uplimit=Dishwasher_On+66+86400*5  IntervalClosedLeft=on  lowlimit=Dishwasher_On+52+86400*5  OutDataTypeStr=boolean
  Switch{,1..2,4} (4 alike) : Switch  Criteria=u2 > Threshold  Threshold=0.5
  Out1 : Outport  VectorParamsAs1DForOutWhenUnconnected=off
  wires:
  Clock/1 -> Gain/1
  Interval Test/1 -> Switch/2
  Constant1/1 -> Switch2/3, Switch/3
  Gain/1 -> Interval Test/1, Interval Test1/1
  Constant3/1 -> Compare To Zero/1
  Constant/1 -> Switch1/1
  Constant2/1 -> Switch1/3
  Compare To Zero/1 -> Switch1/2
  Switch1/1 -> Switch/1
  Interval Test1/1 -> Switch2/2
  Constant6/1 -> Compare To Zero1/1
  Constant4/1 -> Switch4/1
  Constant5/1 -> Switch4/3
  Compare To Zero1/1 -> Switch4/2
  Switch4/1 -> Switch2/1
  Switch/1 -> Add/1
  Switch2/1 -> Add/2
  Add/1 -> Out1/1

== system Microgrid_W/House 5 W1/Light 2/D7 ==
  Add : Sum
  Clock : Clock
  Compare To Zero : simulink/Logic and Bit Operations/Compare To Zero  relop=>  OutDataTypeStr=boolean
  Compare To Zero1 : simulink/Logic and Bit Operations/Compare To Zero  relop=>  OutDataTypeStr=boolean
  Constant : Constant
  Constant1 : Constant  Value=0
  Constant2 : Constant  Value=0
  Constant3 : Constant  Value=Dishwasher_On
  Constant4 : Constant
  Constant5 : Constant  Value=0
  Constant6 : Constant  Value=Dishwasher_On
  Gain : Gain  Gain=t
  Interval Test : simulink/Logic and Bit Operations/Interval Test  IntervalClosedRight=on  uplimit=Dishwasher_On+23+86400*6  IntervalClosedLeft=on  lowlimit=Dishwasher_On+13+86400*6  OutDataTypeStr=boolean
  Interval Test1 : simulink/Logic and Bit Operations/Interval Test  IntervalClosedRight=on  uplimit=Dishwasher_On+66+86400*6  IntervalClosedLeft=on  lowlimit=Dishwasher_On+52+86400*6  OutDataTypeStr=boolean
  Switch{,1..2,4} (4 alike) : Switch  Criteria=u2 > Threshold  Threshold=0.5
  Out1 : Outport  VectorParamsAs1DForOutWhenUnconnected=off
  wires:
  Clock/1 -> Gain/1
  Add/1 -> Out1/1
  Switch2/1 -> Add/2
  Switch/1 -> Add/1
  Switch4/1 -> Switch2/1
  Compare To Zero1/1 -> Switch4/2
  Constant5/1 -> Switch4/3
  Constant4/1 -> Switch4/1
  Constant6/1 -> Compare To Zero1/1
  Interval Test1/1 -> Switch2/2
  Switch1/1 -> Switch/1
  Compare To Zero/1 -> Switch1/2
  Constant2/1 -> Switch1/3
  Constant/1 -> Switch1/1
  Constant3/1 -> Compare To Zero/1
  Gain/1 -> Interval Test1/1, Interval Test/1
  Constant1/1 -> Switch/3, Switch2/3
  Interval Test/1 -> Switch/2

== system Microgrid_W/House 5 W1/Light 2/D8 ==
  Add : Sum  Inputs=+++
  Clock : Clock
  Compare To Zero : simulink/Logic and Bit Operations/Compare To Zero  relop=>  OutDataTypeStr=boolean
  Compare To Zero1 : simulink/Logic and Bit Operations/Compare To Zero  relop=>  OutDataTypeStr=boolean
  Compare To Zero2 : simulink/Logic and Bit Operations/Compare To Zero  relop=>  OutDataTypeStr=boolean
  Constant : Constant
  Constant{1..2,5,8} (4 alike) : Constant  Value=0
  Constant3 : Constant  Value=Dishwasher_On
  Constant4 : Constant
  Constant6 : Constant  Value=Dishwasher_On
  Constant7 : Constant
  Constant9 : Constant  Value=Dishwasher_On
  Gain : Gain  Gain=t
  Interval Test : simulink/Logic and Bit Operations/Interval Test  IntervalClosedRight=on  uplimit=Dishwasher_On+89  IntervalClosedLeft=on  lowlimit=Dishwasher_On+82  OutDataTypeStr=boolean
  Interval Test1 : simulink/Logic and Bit Operations/Interval Test  IntervalClosedRight=on  uplimit=Dishwasher_On+95  IntervalClosedLeft=on  lowlimit=Dishwasher_On+90  OutDataTypeStr=boolean
  Interval Test2 : simulink/Logic and Bit Operations/Interval Test  IntervalClosedRight=on  uplimit=Dishwasher_On+102  IntervalClosedLeft=on  lowlimit=Dishwasher_On+97  OutDataTypeStr=boolean
  Switch{,1..5} (6 alike) : Switch  Criteria=u2 > Threshold  Threshold=0.5
  Out1 : Outport  VectorParamsAs1DForOutWhenUnconnected=off
  wires:
  Clock/1 -> Gain/1
  Add/1 -> Out1/1
  Switch3/1 -> Add/3
  Switch2/1 -> Add/2
  Switch/1 -> Add/1
  Switch5/1 -> Switch3/1
  Switch4/1 -> Switch2/1
  Compare To Zero2/1 -> Switch5/2
  Constant8/1 -> Switch5/3
  Constant7/1 -> Switch5/1
  Constant9/1 -> Compare To Zero2/1
  Compare To Zero1/1 -> Switch4/2
  Constant5/1 -> Switch4/3
  Constant4/1 -> Switch4/1
  Constant6/1 -> Compare To Zero1/1
  Interval Test2/1 -> Switch3/2
  Interval Test1/1 -> Switch2/2
  Switch1/1 -> Switch/1
  Compare To Zero/1 -> Switch1/2
  Constant2/1 -> Switch1/3
  Constant/1 -> Switch1/1
  Constant3/1 -> Compare To Zero/1
  Gain/1 -> Interval Test/1, Interval Test1/1, Interval Test2/1
  Constant1/1 -> Switch/3, Switch2/3, Switch3/3
  Interval Test/1 -> Switch/2

== system Microgrid_W/House 5 W1/Light 2/D9 ==
  Add : Sum  Inputs=+++
  Clock : Clock
  Compare To Zero : simulink/Logic and Bit Operations/Compare To Zero  relop=>  OutDataTypeStr=boolean
  Compare To Zero1 : simulink/Logic and Bit Operations/Compare To Zero  relop=>  OutDataTypeStr=boolean
  Compare To Zero2 : simulink/Logic and Bit Operations/Compare To Zero  relop=>  OutDataTypeStr=boolean
  Constant : Constant
  Constant{1..2,5,8} (4 alike) : Constant  Value=0
  Constant3 : Constant  Value=Dishwasher_On
  Constant4 : Constant
  Constant6 : Constant  Value=Dishwasher_On
  Constant7 : Constant
  Constant9 : Constant  Value=Dishwasher_On
  Gain : Gain  Gain=t
  Interval Test : simulink/Logic and Bit Operations/Interval Test  IntervalClosedRight=on  uplimit=Dishwasher_On+89+86400  IntervalClosedLeft=on  lowlimit=Dishwasher_On+82+86400  OutDataTypeStr=boolean
  Interval Test1 : simulink/Logic and Bit Operations/Interval Test  IntervalClosedRight=on  uplimit=Dishwasher_On+95+86400  IntervalClosedLeft=on  lowlimit=Dishwasher_On+90+86400  OutDataTypeStr=boolean
  Interval Test2 : simulink/Logic and Bit Operations/Interval Test  IntervalClosedRight=on  uplimit=Dishwasher_On+102+86400  IntervalClosedLeft=on  lowlimit=Dishwasher_On+97+86400  OutDataTypeStr=boolean
  Switch{,1..5} (6 alike) : Switch  Criteria=u2 > Threshold  Threshold=0.5
  Out1 : Outport  VectorParamsAs1DForOutWhenUnconnected=off
  wires:
  Clock/1 -> Gain/1
  Interval Test/1 -> Switch/2
  Constant1/1 -> Switch3/3, Switch2/3, Switch/3
  Gain/1 -> Interval Test2/1, Interval Test1/1, Interval Test/1
  Constant3/1 -> Compare To Zero/1
  Constant/1 -> Switch1/1
  Constant2/1 -> Switch1/3
  Compare To Zero/1 -> Switch1/2
  Switch1/1 -> Switch/1
  Interval Test1/1 -> Switch2/2
  Interval Test2/1 -> Switch3/2
  Constant6/1 -> Compare To Zero1/1
  Constant4/1 -> Switch4/1
  Constant5/1 -> Switch4/3
  Compare To Zero1/1 -> Switch4/2
  Constant9/1 -> Compare To Zero2/1
  Constant7/1 -> Switch5/1
  Constant8/1 -> Switch5/3
  Compare To Zero2/1 -> Switch5/2
  Switch4/1 -> Switch2/1
  Switch5/1 -> Switch3/1
  Switch/1 -> Add/1
  Switch2/1 -> Add/2
  Switch3/1 -> Add/3
  Add/1 -> Out1/1

== system Microgrid_W/House 5 W1/Light 4/D1 ==
  Add : Sum
  Clock : Clock
  Constant : Constant
  Constant1 : Constant  Value=0
  Gain : Gain  Gain=t
  Interval Test : simulink/Logic and Bit Operations/Interval Test  IntervalClosedRight=on  uplimit=K_L3_Off_1  IntervalClosedLeft=on  lowlimit=K_L3_On_1  OutDataTypeStr=boolean
  Interval Test1 : simulink/Logic and Bit Operations/Interval Test  IntervalClosedRight=on  uplimit=K_L3_Off_2  IntervalClosedLeft=on  lowlimit=K_L3_On_2  OutDataTypeStr=boolean
  Switch : Switch  Criteria=u2 > Threshold  Threshold=0.5
  Switch1 : Switch  Criteria=u2 > Threshold  Threshold=0.5
  Out1 : Outport  VectorParamsAs1DForOutWhenUnconnected=off
  wires:
  Clock/1 -> Gain/1
  Gain/1 -> Interval Test/1, Interval Test1/1
  Switch1/1 -> Add/2
  Constant/1 -> Switch1/1, Switch/1
  Constant1/1 -> Switch1/3, Switch/3
  Add/1 -> Out1/1
  Interval Test1/1 -> Switch1/2
  Switch/1 -> Add/1
  Interval Test/1 -> Switch/2

== system Microgrid_W/House 5 W1/Light 4/D2 ==
  Add : Sum
  Clock : Clock
  Constant : Constant
  Constant1 : Constant  Value=0
  Gain : Gain  Gain=t
  Interval Test : simulink/Logic and Bit Operations/Interval Test  IntervalClosedRight=on  uplimit=K_L3_Off_1+86400  IntervalClosedLeft=on  lowlimit=K_L3_On_1+86400  OutDataTypeStr=boolean
  Interval Test1 : simulink/Logic and Bit Operations/Interval Test  IntervalClosedRight=on  uplimit=K_L3_Off_2+86400  IntervalClosedLeft=on  lowlimit=K_L3_On_2+86400  OutDataTypeStr=boolean
  Switch : Switch  Criteria=u2 > Threshold  Threshold=0.5
  Switch1 : Switch  Criteria=u2 > Threshold  Threshold=0.5
  Out1 : Outport  VectorParamsAs1DForOutWhenUnconnected=off
  wires:
  Clock/1 -> Gain/1
  Interval Test/1 -> Switch/2
  Switch/1 -> Add/1
  Interval Test1/1 -> Switch1/2
  Add/1 -> Out1/1
  Constant1/1 -> Switch/3, Switch1/3
  Constant/1 -> Switch/1, Switch1/1
  Switch1/1 -> Add/2
  Gain/1 -> Interval Test1/1, Interval Test/1

== system Microgrid_W/House 5 W1/Light 4/D3 ==
  Add : Sum
  Clock : Clock
  Constant : Constant
  Constant1 : Constant  Value=0
  Gain : Gain  Gain=t
  Interval Test : simulink/Logic and Bit Operations/Interval Test  IntervalClosedRight=on  uplimit=K_L3_Off_1+86400*2  IntervalClosedLeft=on  lowlimit=K_L3_On_1+86400*2  OutDataTypeStr=boolean
  Interval Test1 : simulink/Logic and Bit Operations/Interval Test  IntervalClosedRight=on  uplimit=K_L3_Off_2+86400*2  IntervalClosedLeft=on  lowlimit=K_L3_On_2+86400*2  OutDataTypeStr=boolean
  Switch : Switch  Criteria=u2 > Threshold  Threshold=0.5
  Switch1 : Switch  Criteria=u2 > Threshold  Threshold=0.5
  Out1 : Outport  VectorParamsAs1DForOutWhenUnconnected=off
  wires:
  Clock/1 -> Gain/1
  Gain/1 -> Interval Test/1, Interval Test1/1
  Switch1/1 -> Add/2
  Constant/1 -> Switch1/1, Switch/1
  Constant1/1 -> Switch1/3, Switch/3
  Add/1 -> Out1/1
  Interval Test1/1 -> Switch1/2
  Switch/1 -> Add/1
  Interval Test/1 -> Switch/2

== system Microgrid_W/House 5 W1/Light 4/D4 ==
  Add : Sum
  Clock : Clock
  Constant : Constant
  Constant1 : Constant  Value=0
  Gain : Gain  Gain=t
  Interval Test : simulink/Logic and Bit Operations/Interval Test  IntervalClosedRight=on  uplimit=K_L3_Off_1+86400*3  IntervalClosedLeft=on  lowlimit=K_L3_On_1+86400*3  OutDataTypeStr=boolean
  Interval Test1 : simulink/Logic and Bit Operations/Interval Test  IntervalClosedRight=on  uplimit=K_L3_Off_2+86400*3  IntervalClosedLeft=on  lowlimit=K_L3_On_2+86400*3  OutDataTypeStr=boolean
  Switch : Switch  Criteria=u2 > Threshold  Threshold=0.5
  Switch1 : Switch  Criteria=u2 > Threshold  Threshold=0.5
  Out1 : Outport  VectorParamsAs1DForOutWhenUnconnected=off
  wires:
  Clock/1 -> Gain/1
  Interval Test/1 -> Switch/2
  Switch/1 -> Add/1
  Interval Test1/1 -> Switch1/2
  Add/1 -> Out1/1
  Constant1/1 -> Switch/3, Switch1/3
  Constant/1 -> Switch/1, Switch1/1
  Switch1/1 -> Add/2
  Gain/1 -> Interval Test1/1, Interval Test/1

== system Microgrid_W/House 5 W1/Light 4/D5 ==
  Add : Sum
  Clock : Clock
  Constant : Constant
  Constant1 : Constant  Value=0
  Gain : Gain  Gain=t
  Interval Test : simulink/Logic and Bit Operations/Interval Test  IntervalClosedRight=on  uplimit=K_L3_Off_1+86400*4  IntervalClosedLeft=on  lowlimit=K_L3_On_1+86400*4  OutDataTypeStr=boolean
  Interval Test1 : simulink/Logic and Bit Operations/Interval Test  IntervalClosedRight=on  uplimit=K_L3_Off_2+86400*4  IntervalClosedLeft=on  lowlimit=K_L3_On_2+86400*4  OutDataTypeStr=boolean
  Switch : Switch  Criteria=u2 > Threshold  Threshold=0.5
  Switch1 : Switch  Criteria=u2 > Threshold  Threshold=0.5
  Out1 : Outport  VectorParamsAs1DForOutWhenUnconnected=off
  wires:
  Clock/1 -> Gain/1
  Gain/1 -> Interval Test/1, Interval Test1/1
  Switch1/1 -> Add/2
  Constant/1 -> Switch1/1, Switch/1
  Constant1/1 -> Switch1/3, Switch/3
  Add/1 -> Out1/1
  Interval Test1/1 -> Switch1/2
  Switch/1 -> Add/1
  Interval Test/1 -> Switch/2

== system Microgrid_W/House 5 W1/Light 4/D6 ==
  Add : Sum
  Clock : Clock
  Constant : Constant
  Constant1 : Constant  Value=0
  Gain : Gain  Gain=t
  Interval Test : simulink/Logic and Bit Operations/Interval Test  IntervalClosedRight=on  uplimit=K_L3_Off_1+86400*5  IntervalClosedLeft=on  lowlimit=K_L3_On_1+86400*5  OutDataTypeStr=boolean
  Interval Test1 : simulink/Logic and Bit Operations/Interval Test  IntervalClosedRight=on  uplimit=K_L3_Off_2+86400*5  IntervalClosedLeft=on  lowlimit=K_L3_On_2+86400*5  OutDataTypeStr=boolean
  Switch : Switch  Criteria=u2 > Threshold  Threshold=0.5
  Switch1 : Switch  Criteria=u2 > Threshold  Threshold=0.5
  Out1 : Outport  VectorParamsAs1DForOutWhenUnconnected=off
  wires:
  Clock/1 -> Gain/1
  Interval Test/1 -> Switch/2
  Switch/1 -> Add/1
  Interval Test1/1 -> Switch1/2
  Add/1 -> Out1/1
  Constant1/1 -> Switch/3, Switch1/3
  Constant/1 -> Switch/1, Switch1/1
  Switch1/1 -> Add/2
  ? -> Interval Test1/1, Interval Test/1

== system Microgrid_W/House 5 W1/Light 4/D7 ==
  Add : Sum
  Clock : Clock
  Constant : Constant
  Constant1 : Constant  Value=0
  Gain : Gain  Gain=t
  Interval Test : simulink/Logic and Bit Operations/Interval Test  IntervalClosedRight=on  uplimit=K_L3_Off_1+86400*6  IntervalClosedLeft=on  lowlimit=K_L3_On_1+86400*6  OutDataTypeStr=boolean
  Interval Test1 : simulink/Logic and Bit Operations/Interval Test  IntervalClosedRight=on  uplimit=K_L3_Off_2+86400*6  IntervalClosedLeft=on  lowlimit=K_L3_On_2+86400*6  OutDataTypeStr=boolean
  Switch : Switch  Criteria=u2 > Threshold  Threshold=0.5
  Switch1 : Switch  Criteria=u2 > Threshold  Threshold=0.5
  Out1 : Outport  VectorParamsAs1DForOutWhenUnconnected=off
  wires:
  Clock/1 -> Gain/1
  Gain/1 -> Interval Test/1, Interval Test1/1
  Switch1/1 -> Add/2
  Constant/1 -> Switch1/1, Switch/1
  Constant1/1 -> Switch1/3, Switch/3
  Add/1 -> Out1/1
  Interval Test1/1 -> Switch1/2
  Switch/1 -> Add/1
  Interval Test/1 -> Switch/2

== system Microgrid_W/House 5 W1/Light 5/D1 ==
  Clock : Clock
  Constant : Constant
  Constant1 : Constant  Value=0
  Gain : Gain  Gain=t
  Interval Test : simulink/Logic and Bit Operations/Interval Test  IntervalClosedRight=on  uplimit=K_L4_Off_1  IntervalClosedLeft=on  lowlimit=K_L4_On_1  OutDataTypeStr=boolean
  Switch : Switch  Criteria=u2 > Threshold  Threshold=0.5
  Out1 : Outport  VectorParamsAs1DForOutWhenUnconnected=off
  wires:
  Clock/1 -> Gain/1
  Gain/1 -> Interval Test/1
  Constant/1 -> Switch/1
  Constant1/1 -> Switch/3
  Switch/1 -> Out1/1
  Interval Test/1 -> Switch/2

== system Microgrid_W/House 5 W1/Light 5/D2 ==
  Clock : Clock
  Constant : Constant
  Constant1 : Constant  Value=0
  Gain : Gain  Gain=t
  Interval Test : simulink/Logic and Bit Operations/Interval Test  IntervalClosedRight=on  uplimit=K_L4_Off_1+86400  IntervalClosedLeft=on  lowlimit=K_L4_On_1+86400  OutDataTypeStr=boolean
  Switch : Switch  Criteria=u2 > Threshold  Threshold=0.5
  Out1 : Outport  VectorParamsAs1DForOutWhenUnconnected=off
  wires:
  Clock/1 -> Gain/1
  Interval Test/1 -> Switch/2
  Switch/1 -> Out1/1
  Constant1/1 -> Switch/3
  Constant/1 -> Switch/1
  Gain/1 -> Interval Test/1

== system Microgrid_W/House 5 W1/Light 5/D3 ==
  Clock : Clock
  Constant : Constant
  Constant1 : Constant  Value=0
  Gain : Gain  Gain=t
  Interval Test : simulink/Logic and Bit Operations/Interval Test  IntervalClosedRight=on  uplimit=K_L4_Off_1+86400*2  IntervalClosedLeft=on  lowlimit=K_L4_On_1+86400*2  OutDataTypeStr=boolean
  Switch : Switch  Criteria=u2 > Threshold  Threshold=0.5
  Out1 : Outport  VectorParamsAs1DForOutWhenUnconnected=off
  wires:
  Clock/1 -> Gain/1
  Gain/1 -> Interval Test/1
  Constant/1 -> Switch/1
  Constant1/1 -> Switch/3
  Switch/1 -> Out1/1
  Interval Test/1 -> Switch/2

== system Microgrid_W/House 5 W1/Light 5/D4 ==
  Clock : Clock
  Constant : Constant
  Constant1 : Constant  Value=0
  Gain : Gain  Gain=t
  Interval Test : simulink/Logic and Bit Operations/Interval Test  IntervalClosedRight=on  uplimit=K_L4_Off_1+86400*3  IntervalClosedLeft=on  lowlimit=K_L4_On_1+86400*3  OutDataTypeStr=boolean
  Switch : Switch  Criteria=u2 > Threshold  Threshold=0.5
  Out1 : Outport  VectorParamsAs1DForOutWhenUnconnected=off
  wires:
  Clock/1 -> Gain/1
  Interval Test/1 -> Switch/2
  Switch/1 -> Out1/1
  Constant1/1 -> Switch/3
  Constant/1 -> Switch/1
  Gain/1 -> Interval Test/1
